simulink model "tqdtqr_rebuild_V3"  (R2021b)
settings: Solver=VariableStepAuto  StartTime=0.0  StopTime=10.0  RelTol=1e-3
undefined symbols (not defined in the file): ATQD_AfterTqMinGain_X_Deg, ATQD_APSCreepBaseTqD_X_kph, ATQD_APSCreepBaseTqD_Y_Deg, ATQD_APSCreepBaseTqR_X_kph, ATQD_APSCreepBaseTqR_Y_Deg, ATQD_APSCreepIterm_X_kph, ATQD_APSCreepIterm_Y_kph, ATQD_APSCreepPterm_X_kph, ATQD_APSCreepPterm_Y_kph, ATQD_APSDecReq_X_kph, ATQD_APSDecReq_Y_mps2, ATQD_APSDecReqCMD_X_kph, ATQD_APSDecReqTs_X_pct, ATQD_APSDecTimeGain_X_Deg, ATQD_APSDecTimeGain_Y_s, ATQD_APSReqLowSpd_X_Deg, ATQD_AutoHoldReleaseBPS_X_Deg, ATQD_AWDLoadTrqnsGain_X_kg, ATQD_AWDLoadTrqnsGain_Y_pct, ATQD_BOSEnBPSPosn_X_kph, ATQD_BOSMap_X_rpm, ATQD_BOSMap_Y_pct, ATQD_CreepBaseTqD_X_kph, ATQD_CreepBaseTqD_Y_Deg, ATQD_CreepBaseTqR_X_kph, ATQD_CreepBaseTqR_Y_Deg, ATQD_CreepBPSDisPosn_X_Deg, ATQD_CreepBPSDisPosnR_X_Deg, ATQD_CreepBPSEnPosn_X_Deg, ATQD_CreepBPSEnPosnR_X_Deg, ATQD_CreepDeltaTq_X_kph, ATQD_CreepIterm_X_kph, ATQD_CreepIterm_Y_kph, ATQD_CreepItermMaxLimit_X_pct, ATQD_CreepPreloadTime_X_kph, ATQD_CreepPreloadTq_X_kph, ATQD_CreepPreloadTq_Y_s, ATQD_CreepProtTq_X_Deg, ATQD_CreepPterm_X_kph, ATQD_CreepPterm_Y_kph, ATQD_CreepRrTqSpRat_X_rpm, ATQD_CreepRrTqSpRat_Y_Nm, ATQD_CreepTargetSpdD_X_pct, ATQD_CreepTargetSpdR_X_pct, ATQD_CreepUpLimitTq_X_rpm, ATQD_DecIneOPDHoldEnDelay_X_Deg, ATQD_DecIneOPDHoldEnDelay_Y_bar, ATQD_ECOTqMapD_X_rpm, ATQD_ECOTqMapD_Y_pct, ATQD_EMTqMapD_X_rpm, ATQD_EMTqMapD_Y_pct, ATQD_EOPDTqMapDCon_X_rpm, ATQD_EOPDTqMapDCon_Y_Deg, ATQD_EstInitVehWeight_X_c, ATQD_FAfterTqCMDGain_X_rpm, ATQD_FAfterTqCMDGain_Y_pct, ATQD_ForceLowSpd_X_Deg, ATQD_ForcePLimitSpd_X_Deg, ATQD_FrLossMAPLowV_X_rpm, ATQD_FrLossMAPLowV_Y_Nm ... (+949)
libraries: simulink x235, hcu_lib x208, tqr x63, tqd x6
(part 28 of 37)

== system tqdtqr_rebuild_V3/Input_Convert/Signal function/SWC1 SWC2 status/SWC2_Subsystem/Road Speed Limit Convert ==
  note: change units and ouput speed
  note: Calculate speed after offset
  note: Calculate road limit speed
  VINP_ADASSLIFSpdLim_enum : Inport
  VINP_IVIISAOffsetSpd_enum : Inport  Port=2
  VTQD_IVIISAOffsetSpdCHOOSE_flg : Inport  Port=3
  VINP_Distanceunit_flg : Inport  Port=4
  VTQD_ShiftGearPosn_enum : Inport  Port=5
  " 20" : Constant  Value=KTQD_ACCActiveMetSpdLoMPH_mph
  " 30kph" : Constant  Value=KTQD_ACCActiveMetSpdLo_kph
  AND{,1..3} (4 alike) : Logic  AllPortsSameDT=off  OutDataTypeStr=boolean
  Add{,1..3} (4 alike) : Sum  Inputs=+-
  Add4 : Sum
  Constant{,17..18,20} (4 alike) : Constant  Value=0x11  OutDataTypeStr=uint8
  Constant1 : Constant  Value=10  OutDataTypeStr=single
  Constant10 : Constant  Value=15  OutDataTypeStr=single
  Constant11 : Constant  Value=ZERO_FLOAT  OutDataTypeStr=single
  Constant12 : Constant  Value=ENUM_GEARPOSNTOCAN_D  OutDataTypeStr=uint8
  Constant13 : Constant  Value=ZERO_FLOAT  OutDataTypeStr=single
  Constant15 : Constant  Value=ZERO_FLOAT  OutDataTypeStr=single
  Constant16 : Constant  Value=KTQD_SpdLimOffsetOn_flg  OutDataTypeStr=single
  Constant19 : Constant  Value=MPH2KPH  OutDataTypeStr=uint8
  Constant2 : Constant  Value=0xF  OutDataTypeStr=uint8
  Constant21 : Constant  Value=KPH2MPH  OutDataTypeStr=uint8
  Constant22 : Constant  Value=0x0  OutDataTypeStr=uint8
  Constant23 : Constant  Value=0x6  OutDataTypeStr=uint8
  Constant24 : Constant  Value=0x7  OutDataTypeStr=uint8
  Constant25 : Constant  Value=0x8  OutDataTypeStr=uint8
  Constant26 : Constant  Value=0xC  OutDataTypeStr=uint8
  Constant{3,7..9} (4 alike) : Constant  Value=5  OutDataTypeStr=single
  Constant4 : Constant  Value=0x0  OutDataTypeStr=uint8
  Constant5 : Constant  Value=0x9  OutDataTypeStr=uint8
  Constant6 : Constant  Value=0x9  OutDataTypeStr=uint8
  Data Type Conversion{,1..3} (4 alike) : DataTypeConversion  OutDataTypeStr=single
  Delay : Delay  DelayLength=1
      settings: AttributesFormatString=%<InitialCondition>
  Divide : Product  Inputs=**
  Divide1 : Product  Inputs=**
  Equal : RelationalOperator  Operator=~=  OutDataTypeStr=boolean  RndMeth=Simplest
  Equal1 : RelationalOperator  Operator===  OutDataTypeStr=boolean  RndMeth=Simplest
  Max : MinMax  Function=max  Inputs=2
  NOT : Logic  Operator=NOT  AllPortsSameDT=off  OutDataTypeStr=boolean
  NOT1 : Logic  Operator=NOT  AllPortsSameDT=off  OutDataTypeStr=boolean
  OR : Logic  Operator=OR  Inputs=5  AllPortsSameDT=off  OutDataTypeStr=boolean
  Product{,1..3} (4 alike) : Product
  Relational Operator{,1,3..5,10} (6 alike) : RelationalOperator  OutDataTypeStr=boolean  RndMeth=Simplest
  Relational Operator{6..9} (4 alike) : RelationalOperator  Operator===  OutDataTypeStr=boolean  RndMeth=Simplest
  Switch{,1..9} (10 alike) : Switch  Criteria=u2 ~= 0
      settings: AttributesFormatString=%<Criteria>
  VTQD_RoadSpdLim_raw32 : Outport
  wires:
  Relational Operator10/1 -> OR/5
  Relational Operator9/1 -> OR/4
  Relational Operator8/1 -> OR/3
  Relational Operator7/1 -> OR/2
  Relational Operator6/1 -> OR/1
  [VINP_IVIISAOffsetSpd_enum] -> Relational Operator10/1
  Constant26/1 -> Relational Operator10/2
  Constant25/1 -> Relational Operator9/2
  [VINP_IVIISAOffsetSpd_enum] -> Relational Operator9/1
  [VINP_IVIISAOffsetSpd_enum] -> Relational Operator8/1
  Constant24/1 -> Relational Operator8/2
  Constant23/1 -> Relational Operator7/2
  [VINP_IVIISAOffsetSpd_enum] -> Relational Operator7/1
  [VINP_IVIISAOffsetSpd_enum] -> Relational Operator6/1
  Constant22/1 -> Relational Operator6/2
  [VTQD_SpdLimAftOffset_raw32] -> Switch9/3
  Divide1/1 -> Switch9/1
  [VTQD_SpdLimAftOffset_raw32] -> Divide1/1
  Constant21/1 -> Divide1/2
  NOT1/1 -> AND3/2
  Switch9/1 -> Switch8/3
  Constant20/1 -> Relational Operator5/2
  [VINP_ADASSLIFSpdLim_enum] -> Relational Operator5/1
  Relational Operator5/1 -> NOT1/1
  [VINP_Distanceunit_flg] -> AND3/1
  AND3/1 -> Switch9/2
  Constant19/1 -> Divide/2
  Divide/1 -> Switch8/1
  [VTQD_SpdLimAftOffset_raw32] -> Divide/1
  NOT/1 -> AND2/1
  Switch8/1 -> Switch7/3
  Constant18/1 -> Relational Operator4/2
  [VINP_ADASSLIFSpdLim_enum] -> Relational Operator4/1
  Relational Operator4/1 -> AND2/2
  [VINP_Distanceunit_flg] -> NOT/1
  AND2/1 -> Switch8/2
  [VTQD_SpdLimAftOffset_raw32] -> Switch7/1
  Switch7/1 -> Max/2
  AND1/1 -> Switch7/2
  [VINP_Distanceunit_flg] -> AND1/1
  Relational Operator3/1 -> AND1/2
  [VINP_ADASSLIFSpdLim_enum] -> Relational Operator3/1
  Constant17/1 -> Relational Operator3/2
  Constant16/1 -> AND/2
  AND/1 -> Switch3/2
  Constant15/1 -> Switch6/1
  OR/1 -> Switch6/2
  [VTQD_CalRoadSpdLimOffSet_c] -> Switch6/3
  [VTQD_ShiftGearPosn_enum] -> Equal1/1
  VTQD_ShiftGearPosn_enum/1 -> [VTQD_ShiftGearPosn_enum]
  Constant13/1 -> Switch5/3
  Switch1/1 -> Switch5/1
  Constant12/1 -> Equal1/2
  Equal1/1 -> Switch5/2
  [VINP_ADASSLIFSpdLim_enum] -> Equal/1
  Add4/1 -> [VTQD_SpdLimAftOffset_raw32]  "VTQD_SpdLimAftOffset_raw32"
  Max/1 -> [VTQD_RoadSpdLim_raw32]  "VTQD_RoadSpdLim_raw32"
  Switch4/1 -> Max/1
  Delay/1 -> Switch1/3
  VINP_Distanceunit_flg/1 -> [VINP_Distanceunit_flg]
  [VINP_Distanceunit_flg] -> Switch4/2
  " 30kph"/1 -> Switch4/3
  " 20"/1 -> Switch4/1
  [VTQD_IVIISAOffsetSpdCHOOSE_flg] -> AND/1
  [VTQD_RoadSpdLim_raw32] -> VTQD_RoadSpdLim_raw32/1
  [VTQD_CalRoadSpdLim_raw32] -> Add4/1
  Switch6/1 -> Add4/2
  Switch3/1 -> [VTQD_CalRoadSpdLimOffSet_c]  "VTQD_CalRoadSpdLimOffSet_c"
  Constant11/1 -> Switch3/3
  Switch2/1 -> Switch3/1
  VTQD_IVIISAOffsetSpdCHOOSE_flg/1 -> [VTQD_IVIISAOffsetSpdCHOOSE_flg]
  Add2/1 -> Switch2/1
  Add3/1 -> Switch2/3
  Product3/1 -> Add3/1
  Constant10/1 -> Add3/2
  Data Type Conversion3/1 -> Product3/1
  Constant9/1 -> Product3/2
  [VINP_IVIISAOffsetSpd_enum] -> Data Type Conversion3/1
  Constant8/1 -> Add2/2
  Product2/1 -> Add2/1
  Constant7/1 -> Product2/2
  Add1/1 -> Data Type Conversion2/1
  Constant6/1 -> Add1/2
  [VINP_IVIISAOffsetSpd_enum] -> Add1/1
  Data Type Conversion2/1 -> Product2/1
  Relational Operator1/1 -> Switch2/2
  Constant5/1 -> Relational Operator1/2
  [VINP_IVIISAOffsetSpd_enum] -> Relational Operator1/1
  Switch5/1 -> Delay/1, [VTQD_CalRoadSpdLim_raw32]  "VTQD_CalRoadSpdLim_raw32"
  Switch/1 -> Switch1/1
  Constant4/1 -> Equal/2
  Equal/1 -> Switch1/2
  Data Type Conversion1/1 -> Product1/1
  Add/1 -> Data Type Conversion1/1
  Constant3/1 -> Product1/2
  Product1/1 -> Switch/1
  Constant2/1 -> Add/2
  [VINP_ADASSLIFSpdLim_enum] -> Add/1
  Product/1 -> Switch/3
  Constant1/1 -> Product/2
  Data Type Conversion/1 -> Product/1
  [VINP_ADASSLIFSpdLim_enum] -> Data Type Conversion/1
  Constant/1 -> Relational Operator/2
  Relational Operator/1 -> Switch/2
  [VINP_ADASSLIFSpdLim_enum] -> Relational Operator/1
  VINP_IVIISAOffsetSpd_enum/1 -> [VINP_IVIISAOffsetSpd_enum]
  VINP_ADASSLIFSpdLim_enum/1 -> [VINP_ADASSLIFSpdLim_enum]

== system tqdtqr_rebuild_V3/Input_Convert/Signal function/SWC1 SWC2 status/SWC2_Subsystem/Speed Setting Mode ==
  note: Ctrl Mode -> speed(ACC/CC/MSA/ISA)
  note: Ctrl Mode -> OUTPUT SET SPEED
  note: Check PWRSTA and DRIVE GEAR GOOD
  note: INPUT Signal
  note: Botton logic
  VPMM_PowerSta_enum : Inport
  VTQD_ShiftGearPosn_enum : Inport  Port=2
  VTQD_SpdCtrlMode_enum : Inport  Port=3
  VINP_ADASACCSta_enum : Inport  Port=4
  VVMC_CCCtrlSta_enum : Inport  Port=5
  VVMC_MSACtrlSta_enum : Inport  Port=6
  VINP_ADASSLIFSpdLim_enum : Inport  Port=7
  VTQD_SWC2ScrollUpSta_flg : Inport  Port=8
  VTQD_SWC2ScrollDownSta_flg : Inport  Port=9
  task_time_s : Inport  Port=10
  VVMC_LVDAACCStatusInformation_flg : Inport  Port=11
  VTQD_SpdLim4SetSpd_raw32 : Inport  Port=12
  VINP_Distanceunit_flg : Inport  Port=13
  VINP_SmartEcoModeSW_flg : Inport  Port=14
  VINP_IVIACCAdaptiveSta_flg : Inport  Port=15
  VTQD_Set2MeterSpd_flg : Inport  Port=16
  VTQD_SetRoadSpdLim_flg : Inport  Port=17
  VTQD_LScrollPressShort_flg : Inport  Port=18
  VVMC_MeterIndSpeed_raw32 : Inport  Port=19
  ACC Speed Setting ON : Subsystem  TreatAsAtomicUnit=on
  AND{1..5} (5 alike) : Logic  AllPortsSameDT=off  OutDataTypeStr=boolean
  CC Speed Setting ON : Subsystem  TreatAsAtomicUnit=on
  Constant : Constant  Value=ZERO_INT
  Constant1 : Constant  Value=ENUM_SPDCTRLMODE_CC
  Constant10 : Constant  Value=ENUM_SPDCTRLMODE_ISA
  Constant11 : Constant  Value=ENUM_SPDCTRLMODE_OFF
  Constant12 : Constant  Value=KTQD_SetSpdDeltaLongFit_kph
  Constant13 : Constant  Value=ZERO_INT
  Constant2 : Constant  Value=ENUM_POWERSTA_READY
  Constant20 : Constant  Value=KTQD_SpdCtrlModeChgHoldTime_s
  Constant21 : Constant  Value=KTQD_SCPMemSpdTest_flg
  Constant3 : Constant  Value=ENUM_SPDCTRLMODE_ACC
  Constant4 : Constant  Value=ENUM_GEARPOSNTOCAN_D
  Constant5 : Constant  Value=ENUM_SPDCTRLMODE_MSA
  Constant6 : Constant  Value=ENUM_SPDCTRLMODE_ISA
  Constant7 : Constant  Value=ENUM_SPDCTRLMODE_ACC
  Constant8 : Constant  Value=ENUM_SPDCTRLMODE_CC
  Constant9 : Constant  Value=ENUM_SPDCTRLMODE_MSA
  Data Type Conversion : DataTypeConversion  OutDataTypeStr=uint8
  Delay : Delay  DelayLength=1
  Delay Enable : hcu_lib/Basic_Blocks/DelayEnable
  Detect Change : simulink/Logic and Bit Operations/Detect Change  vinit=boolean(0)  OutDataTypeStr=boolean
  Detect Change1 : simulink/Logic and Bit Operations/Detect Change  vinit=boolean(0)  OutDataTypeStr=boolean
  Else Speed Setting On : Subsystem  TreatAsAtomicUnit=on
  Equal{1..11} (11 alike) : RelationalOperator  Operator===  OutDataTypeStr=boolean  RndMeth=Simplest
  ISA Speed Setting ON : Subsystem  TreatAsAtomicUnit=on
  If : If  NumInputs=4  IfExpression=u1 ~= 0  ElseIfExpressions=u2 ~= 0, u3~= 0, u4~= 0
  MSA Speed Setting ON : Subsystem  TreatAsAtomicUnit=on
  Rem : Math  Operator=rem  SaturateOnIntegerOverflow=on
  SR_Latch1 : hcu_lib/Basic_Blocks/SR_Latch
  SR_Latch7 : hcu_lib/Basic_Blocks/SR_Latch
  SWC2ScrollDownSta : Subsystem
  SWC2ScrollUpSta : Subsystem
  Switch{,1..4,8} (6 alike) : Switch  Criteria=u2 ~= 0
      settings: AttributesFormatString=%<Criteria>
  Unit Delay : UnitDelay  InitialCondition=single(0)  SampleTime=-1  HasFrameUpgradeWarning=on
      settings: AttributesFormatString=%<InitialCondition>
  Unit Delay1 : UnitDelay  SampleTime=-1  HasFrameUpgradeWarning=on
  Unit Delay2 : UnitDelay  InitialCondition=boolean(0)  SampleTime=-1  HasFrameUpgradeWarning=on
      settings: AttributesFormatString=%<InitialCondition>
  Unit Delay3 : UnitDelay  InitialCondition=single(0.0)  SampleTime=-1  HasFrameUpgradeWarning=on
      settings: AttributesFormatString=%<InitialCondition>
  VTQD_SetSpd_kph : Outport
  VTQD_SWC2ScrollUpSta_enum : Outport  Port=2
  wires:
  AND4/1 -> Switch8/2
  Constant21/1 -> AND4/2
  SR_Latch1/1 -> AND4/1
  Detect Change1/1 -> SR_Latch1/1
  [VTQD_SpdCtrlMode_enum] -> Detect Change1/1
  Unit Delay3/1 -> Switch8/1
  [VTQD_SetSpd_kph] -> Unit Delay3/1
  Switch/1 -> Switch8/3
  Unit Delay2/1 -> SR_Latch7/2
  SR_Latch7/1 -> Delay Enable/1
  Detect Change/1 -> SR_Latch7/1
  Delay Enable/1 -> Unit Delay2/1, SR_Latch1/2
  Constant20/1 -> Delay Enable/2
  [task_time_s] -> Delay Enable/3
  [VTQD_SpdCtrlMode_enum] -> Detect Change/1
  [VTQD_SetSpd_kph] -> Unit Delay1/1
  Unit Delay1/1 -> MSA Speed Setting ON/13(VTQD_LastSetSpd_kph)
  Unit Delay/1 -> ACC Speed Setting ON/16(VTQD_LastSetSpd_kph)
  [VTQD_SetSpd_kph] -> Unit Delay/1
  [VTQD_SWC2ScrollUpSta_flg] -> ACC Speed Setting ON/15(VTQD_SWC2ScrollUpSta_flg)
  [VTQD_SWC2ScrollDownSta_flg] -> ACC Speed Setting ON/14(VTQD_SWC2ScrollDownSta_flg)
  [VVMC_LVDAACCStatusInformation_flg] -> ACC Speed Setting ON/3(VVMC_LVDAACCStatusInformation_flg)
  VVMC_LVDAACCStatusInformation_flg/1 -> [VVMC_LVDAACCStatusInformation_flg]
  [VVMC_MeterIndSpeed_raw32] -> MSA Speed Setting ON/12(VVMC_MeterIndSpeed_raw32)
  [VVMC_MeterIndSpeed_raw32] -> ACC Speed Setting ON/13(VVMC_MeterIndSpeed_raw32)
  VVMC_MeterIndSpeed_raw32/1 -> [VVMC_MeterIndSpeed_raw32]
  [VTQD_LScrollPressShort_flg] -> MSA Speed Setting ON/11(VTQD_LScrollPressShort_flg)
  [VINP_ADASSLIFSpdLim_enum] -> MSA Speed Setting ON/10(VINP_ADASSLIFSpdLim_enum)
  [VTQD_SetRoadSpdLim_flg] -> MSA Speed Setting ON/9(VTQD_SetRoadSpdLim_flg)
  [VTQD_Set2MeterSpd_flg] -> MSA Speed Setting ON/8(VTQD_Set2MeterSpd_flg)
  [VINP_IVIACCAdaptiveSta_flg] -> MSA Speed Setting ON/7(VINP_IVIACCAdaptiveSta_flg)
  VTQD_LScrollPressShort_flg/1 -> [VTQD_LScrollPressShort_flg]
  VTQD_SetRoadSpdLim_flg/1 -> [VTQD_SetRoadSpdLim_flg]
  VTQD_Set2MeterSpd_flg/1 -> [VTQD_Set2MeterSpd_flg]
  [VINP_IVIACCAdaptiveSta_flg] -> ACC Speed Setting ON/8(VINP_IVIACCAdaptiveSta_flg)
  [VTQD_LScrollPressShort_flg] -> ACC Speed Setting ON/12(VTQD_LScrollPressShort_flg)
  [VINP_ADASSLIFSpdLim_enum] -> ACC Speed Setting ON/11(VINP_ADASSLIFSpdLim_enum)
  [VTQD_SetRoadSpdLim_flg] -> ACC Speed Setting ON/10(VTQD_SetRoadSpdLim_flg)
  [VTQD_Set2MeterSpd_flg] -> ACC Speed Setting ON/9(VTQD_Set2MeterSpd_flg)
  VINP_IVIACCAdaptiveSta_flg/1 -> [VINP_IVIACCAdaptiveSta_flg]
  [VINP_SmartEcoModeSW_flg] -> ISA Speed Setting ON/2(VINP_SmartEcoModeSW_flg)
  [VINP_SmartEcoModeSW_flg] -> MSA Speed Setting ON/6(VINP_SmartEcoModeSW_flg)
  [VINP_SmartEcoModeSW_flg] -> CC Speed Setting ON/7(VINP_SmartEcoModeSW_flg)
  [VINP_SmartEcoModeSW_flg] -> ACC Speed Setting ON/7(VINP_SmartEcoModeSW_flg)
  VINP_SmartEcoModeSW_flg/1 -> [VINP_SmartEcoModeSW_flg]
  [VTQD_SWC2ScrollDownSta_enum] -> MSA Speed Setting ON/3("VTQD_SWC2ScrollDownSta_enum  ")
  [VTQD_SWC2ScrollUpSta_enum] -> MSA Speed Setting ON/2("VTQD_SWC2ScrollUpSta_enum  ")
  [VTQD_SWC2ScrollUpSta_enum] -> ACC Speed Setting ON/1(VTQD_SWC2ScrollUpSta_enum)
  [VTQD_SWC2ScrollDownSta_enum] -> ACC Speed Setting ON/2(VTQD_SWC2ScrollDownSta_enum)
  [VINP_Distanceunit_flg] -> MSA Speed Setting ON/5(VINP_Distanceunit_flg)
  [VINP_Distanceunit_flg] -> CC Speed Setting ON/6(VINP_Distanceunit_flg)
  [VINP_Distanceunit_flg] -> ACC Speed Setting ON/6(VINP_Distanceunit_flg)
  VINP_Distanceunit_flg/1 -> [VINP_Distanceunit_flg]
  VTQD_SpdLim4SetSpd_raw32/1 -> [VTQD_SpdLim4SetSpd_raw32]
  ACC Speed Setting ON/1(VTQD_ACCSetSpd_kph) -> [VTQD_ACCSetSpd_kph]  "VTQD_SWC2ACCSetSpd_kph"
  [VTQD_SpdLim4SetSpd_raw32] -> ACC Speed Setting ON/4(VTQD_SpdLim4SetSpd_raw32)
  [VINP_ADASACCSta_enum] -> ACC Speed Setting ON/5(VINP_ADASACCSta_enum)
  [VTQD_ElseSetSpd_kph] -> Switch4/3
  Else Speed Setting On/1(Out) -> [VTQD_ElseSetSpd_kph]
  Constant13/1 -> Else Speed Setting On/1(In)
  [VTQD_SpdLim4SetSpd_raw32] -> MSA Speed Setting ON/4(VTQD_SpdLim4SetSpd_raw32)
  [VTQD_SpdLim4SetSpd_raw32] -> CC Speed Setting ON/4(VTQD_SpdLim4SetSpd_raw32)
  [VTQD_SetSpdDeltaLongFit_kph] -> CC Speed Setting ON/5(VTQD_SetSpdDeltaLongFit_kph)
  Constant12/1 -> Rem/2
  Delay/1 -> Rem/1
  [VTQD_SetSpd_kph] -> Delay/1
  Data Type Conversion/1 -> [VTQD_SetSpdDeltaLongFit_kph]  "VTQD_SetSpdDeltaLongFit_kph"
  Rem/1 -> Data Type Conversion/1
  [task_time_s] -> SWC2ScrollUpSta/2(task_time_s)
  SWC2ScrollDownSta/1(OUTPUT) -> [VTQD_SWC2ScrollDownSta_enum]  "VTQD_SWC2ScrollDownSta_enum"
  [VTQD_SWC2ScrollDownSta_flg] -> SWC2ScrollDownSta/1(INPUT)
  [task_time_s] -> SWC2ScrollDownSta/2(task_time_s)
  SWC2ScrollUpSta/1(OUTPUT) -> [VTQD_SWC2ScrollUpSta_enum]  "VTQD_SWC2ScrollUpSta_enum"
  [VTQD_SWC2ScrollUpSta_flg] -> SWC2ScrollUpSta/1(INPUT)
  [VINP_ADASSLIFSpdLim_enum] -> ISA Speed Setting ON/1(VINP_ADASSLIFSpdLim_enum)
  VPMM_PowerSta_enum/1 -> [VPMM_PowerSta_enum]
  VTQD_ShiftGearPosn_enum/1 -> [VTQD_ShiftGearPosn_enum]
  [VTQD_PwrstaANDGearRdy_flg] -> AND1/1
  VTQD_SpdCtrlMode_enum/1 -> [VTQD_SpdCtrlMode_enum]
  If/1 -> ACC Speed Setting ON/Action
  [VTQD_SpdCtrlMode_enum] -> Equal3/1
  Constant3/1 -> Equal3/2
  Equal3/1 -> AND1/2
  AND1/1 -> If/1
  Equal4/1 -> AND2/2
  Equal2/1 -> AND2/1
  Constant4/1 -> Equal4/2
  [VTQD_ShiftGearPosn_enum] -> Equal4/1
  Constant2/1 -> Equal2/2
  [VPMM_PowerSta_enum] -> Equal2/1
  AND2/1 -> [VTQD_PwrstaANDGearRdy_flg]  "VTQD_PwrstaANDGearRdy_flg"
  Equal1/1 -> AND3/2
  Constant1/1 -> Equal1/2
  [VTQD_SpdCtrlMode_enum] -> Equal1/1
  [VTQD_PwrstaANDGearRdy_flg] -> AND3/1
  AND3/1 -> If/2
  VTQD_SWC2ScrollUpSta_flg/1 -> [VTQD_SWC2ScrollUpSta_flg]
  VTQD_SWC2ScrollDownSta_flg/1 -> [VTQD_SWC2ScrollDownSta_flg]
  VINP_ADASACCSta_enum/1 -> [VINP_ADASACCSta_enum]
  [VVMC_CCCtrlSta_enum] -> CC Speed Setting ON/1(VVMC_CCCtrlSta_enum)
  [VTQD_SWC2ScrollUpSta_enum] -> CC Speed Setting ON/2("VTQD_SWCResUpPress_enum  ")
  [VTQD_SWC2ScrollDownSta_enum] -> CC Speed Setting ON/3("VTQD_SWCSetDownPress_enum  ")
  If/2 -> CC Speed Setting ON/Action
  [VVMC_MSACtrlSta_enum] -> MSA Speed Setting ON/1(VVMC_MSACrlSta_enum)
  If/3 -> MSA Speed Setting ON/Action
  [VTQD_SpdCtrlMode_enum] -> Equal5/1
  Constant5/1 -> Equal5/2
  Equal5/1 -> If/3
  VVMC_MSACtrlSta_enum/1 -> [VVMC_MSACtrlSta_enum]
  Equal6/1 -> AND5/2
  Constant6/1 -> Equal6/2
  [VTQD_SpdCtrlMode_enum] -> Equal6/1
  [VTQD_PwrstaANDGearRdy_flg] -> AND5/1
  AND5/1 -> If/4
  If/4 -> ISA Speed Setting ON/Action
  If/5 -> Else Speed Setting On/Action
  ISA Speed Setting ON/1(VTQD_ISASetSpd_kph) -> [VTQD_ISASetSpd_kph]  "VTQD_SWC2ISASetSpd_kph"
  Constant7/1 -> Equal7/2
  [VTQD_SpdCtrlMode_enum] -> Equal7/1
  Equal7/1 -> Switch/2
  [VTQD_ACCSetSpd_kph] -> Switch/1
  [VTQD_CCSetSpd_kph] -> Switch1/1
  Equal8/1 -> Switch1/2
  [VTQD_SpdCtrlMode_enum] -> Equal8/1
  Constant8/1 -> Equal8/2
  Switch1/1 -> Switch/3
  Constant9/1 -> Equal9/2
  [VTQD_SpdCtrlMode_enum] -> Equal9/1
  Equal9/1 -> Switch2/2
  [VTQD_MSASetSpd_kph] -> Switch2/1
  Switch2/1 -> Switch1/3
  [VTQD_ISASetSpd_kph] -> Switch3/1
  Equal10/1 -> Switch3/2
  [VTQD_SpdCtrlMode_enum] -> Equal10/1
  Constant10/1 -> Equal10/2
  Switch3/1 -> Switch2/3
  Constant11/1 -> Equal11/2
  [VTQD_SpdCtrlMode_enum] -> Equal11/1
  Equal11/1 -> Switch4/2
  Switch4/1 -> Switch3/3
  Constant/1 -> Switch4/1
  Switch8/1 -> [VTQD_SetSpd_kph]  "VTQD_SetSpd_kph"
  task_time_s/1 -> [task_time_s]
  VINP_ADASSLIFSpdLim_enum/1 -> [VINP_ADASSLIFSpdLim_enum]
  VVMC_CCCtrlSta_enum/1 -> [VVMC_CCCtrlSta_enum]
  CC Speed Setting ON/1(VTQD_CCSetSpd_kph) -> [VTQD_CCSetSpd_kph]  "VTQD_SWC2CCSetSpd_kph"
  MSA Speed Setting ON/1(VSCP_MSASetSpd_kph) -> [VTQD_MSASetSpd_kph]  "VTQD_SWC2MSASetSpd_kph"
  [VTQD_SWC2ScrollUpSta_enum] -> VTQD_SWC2ScrollUpSta_enum/1
  [VTQD_SetSpd_kph] -> VTQD_SetSpd_kph/1

== system tqdtqr_rebuild_V3/Input_Convert/Signal function/SWC1 SWC2 status/SWC2_Subsystem/VTQD_IVIISAOffsetSpdCHOOSE_flg ==
  VTQD_IVIISAOffsetSpd_enum : Inport
  Constant : Constant  Value=ENUM_IVIISAOFFSETSPD_MIUNS10KPH
  Constant1 : Constant  Value=ENUM_IVIISAOFFSETSPD_MIUNS5KPH
  Constant2 : Constant  Value=ENUM_IVIISAOFFSETSPD_0KPH
  Constant3 : Constant  Value=ENUM_IVIISAOFFSETSPD_PLUS5KPH
  Constant4 : Constant  Value=ENUM_IVIISAOFFSETSPD_PLUS10KPH
  Constant5 : Constant  Value=ENUM_IVIISAOFFSETSPD_MIUNS5MPH
  Constant6 : Constant  Value=ENUM_IVIISAOFFSETSPD_0MPH
  Constant7 : Constant  Value=ENUM_IVIISAOFFSETSPD_PLUS5MPH
  Constant8 : Constant  Value=TRUE
  Constant9 : Constant  Value=FALSE
  Equal{,1..7} (8 alike) : RelationalOperator  Operator===  OutDataTypeStr=boolean  RndMeth=Simplest
  OR : Logic  Operator=OR  Inputs=8  AllPortsSameDT=off  OutDataTypeStr=boolean
  Switch : Switch  Criteria=u2 ~= 0
      settings: AttributesFormatString=%<Criteria>
  VTQD_IVIISAOffsetSpdCHOOSE_flg : Outport
  wires:
  [VTQD_IVIISAOffsetSpd_enum] -> Equal3/1
  [VTQD_IVIISAOffsetSpd_enum] -> Equal7/1
  [VTQD_IVIISAOffsetSpd_enum] -> Equal5/1
  [VTQD_IVIISAOffsetSpd_enum] -> Equal6/1
  [VTQD_IVIISAOffsetSpd_enum] -> Equal4/1
  [VTQD_IVIISAOffsetSpd_enum] -> Equal2/1
  [VTQD_IVIISAOffsetSpd_enum] -> Equal1/1
  Switch/1 -> VTQD_IVIISAOffsetSpdCHOOSE_flg/1  "VTQD_IVIISAOffsetSpdCHOOSE_flg"
  Constant9/1 -> Switch/3
  Constant8/1 -> Switch/1
  OR/1 -> Switch/2
  Equal7/1 -> OR/8
  Constant7/1 -> Equal7/2
  Constant6/1 -> Equal6/2
  Equal6/1 -> OR/7
  Constant3/1 -> Equal3/2
  Equal3/1 -> OR/4
  Constant4/1 -> Equal4/2
  Equal4/1 -> OR/5
  Equal5/1 -> OR/6
  Constant5/1 -> Equal5/2
  Constant2/1 -> Equal2/2
  Equal2/1 -> OR/3
  Equal1/1 -> OR/2
  Constant1/1 -> Equal1/2
  Equal/1 -> OR/1
  Constant/1 -> Equal/2
  VTQD_IVIISAOffsetSpd_enum/1 -> [VTQD_IVIISAOffsetSpd_enum]
  [VTQD_IVIISAOffsetSpd_enum] -> Equal/1

== system tqdtqr_rebuild_V3/Input_Convert/Signal function/SWC1 SWC2 status/SWC_Subsystem/SpdCtrlBotton Behavior ==
  note: Long press or Short press
  note: If press time more then Long press's limit then go Long press only. Else go short press only. Else if no press.
  SWC_ACC_Sta : Inport
  TASK_TIME : Inport  Port=2
  AND : Logic  AllPortsSameDT=off  OutDataTypeStr=boolean
  Constant10 : Constant  Value=FALSE
  Constant3 : Constant  Value=KTQD_SpdModeShortPLim_s
  Constant7 : Constant  Value=FALSE
  Default 3 sec : Constant  Value=KTQD_SpdModeLongPLim_s
  DelayEnable_LONG_PRESS : hcu_lib/Basic_Blocks/DelayEnable
  DelayEnable_SHORT_PRESS : hcu_lib/Basic_Blocks/DelayEnable
  Detect Decrease1 : simulink/Logic and Bit Operations/Detect Decrease  vinit=boolean(0)  OutDataTypeStr=boolean
  Detect Decrease2 : simulink/Logic and Bit Operations/Detect Decrease  vinit=boolean(0)  OutDataTypeStr=boolean
  Detect Increase : simulink/Logic and Bit Operations/Detect Increase  vinit=boolean(0)  OutDataTypeStr=boolean
  Switch1 : Switch  Criteria=u2 > Threshold
      settings: AttributesFormatString=%<Criteria>
  Switch2 : Switch  Criteria=u2 ~= 0
      settings: AttributesFormatString=%<Criteria>
  VTQD_SpdCtrlShortP_flg : Outport
  "VTQD_SpdCtrlLongP_flg\t" : Outport  Port=2
  wires:
  TASK_TIME/1 -> [TASK_TIME]
  Switch1/1 -> [Long_press]
  Detect Decrease2/1 -> [Short_press_falling_Edge]
  Detect Decrease1/1 -> AND/2
  SWC_ACC_Sta/1 -> [SWC_ACC_Sta]
  Switch2/1 -> VTQD_SpdCtrlShortP_flg/1
  AND/1 -> Switch2/2
  [SWC_ACC_Sta] -> DelayEnable_LONG_PRESS/1, DelayEnable_SHORT_PRESS/1
  [Short_press_falling_Edge] -> Switch2/3
  Constant10/1 -> Switch2/1
  [Long_press] -> Detect Increase/1, Detect Decrease1/1
  [Short_press_falling_Edge] -> AND/1
  DelayEnable_LONG_PRESS/1 -> Switch1/2, Switch1/1
  Constant7/1 -> Switch1/3
  DelayEnable_SHORT_PRESS/1 -> Detect Decrease2/1
  Constant3/1 -> DelayEnable_SHORT_PRESS/2
  [TASK_TIME] -> DelayEnable_SHORT_PRESS/3
  Default 3 sec/1 -> DelayEnable_LONG_PRESS/2
  [TASK_TIME] -> DelayEnable_LONG_PRESS/3
  Detect Increase/1 -> "VTQD_SpdCtrlLongP_flg\t"/1

== system tqdtqr_rebuild_V3/Input_Convert/Signal function/SWC1 SWC2 status/SWC_Subsystem/Speed Setting Mode ==
  note: CtrlMode -> Calculate speed(ACC/CC/MSA/ISA)
  note: CtrlMode -> OUTPUT SET SPEED
  note: Check PWRSTA and DRIVE GEAR GOOD
  note: INPUT Signal
  note: Botton logic(long/short press)
  VPMM_PowerSta_enum : Inport
  VTQD_ShiftGearPosn_enum : Inport  Port=2
  VTQD_SpdCtrlMode_enum : Inport  Port=3
  VINP_ADASACCSta_enum : Inport  Port=4
  VVMC_CCCtrlSta_enum : Inport  Port=5
  VVMC_MSACtrlSta_enum : Inport  Port=6
  VINP_ADASVehSpdLim_kph : Inport  Port=7
  VTQD_SWCResUpSta_flg : Inport  Port=8
  VTQD_SWCSetDownSta_flg : Inport  Port=9
  task_time_s : Inport  Port=10
  VVMC_LVDAACCStatusInformation_flg : Inport  Port=11
  VVMC_ACCObjDist_m : Inport  Port=12
  VVMC_MeterIndSpeed_raw32 : Inport  Port=13
  VINP_Distanceunit_flg : Inport  Port=14
  VINP_SmartEcoModeSW_flg : Inport  Port=15
  VVMC_SetACCDisableAPS_flg : Inport  Port=16
  ACC Speed Setting ON : Subsystem  TreatAsAtomicUnit=on
  AND{1..5} (5 alike) : Logic  AllPortsSameDT=off  OutDataTypeStr=boolean
  CC Speed Setting ON : Subsystem  TreatAsAtomicUnit=on
  Constant : Constant  Value=ZERO_INT
  Constant1 : Constant  Value=ENUM_SPDCTRLMODE_CC
  Constant10 : Constant  Value=ENUM_SPDCTRLMODE_ISA
  Constant11 : Constant  Value=ENUM_SPDCTRLMODE_OFF
  Constant12 : Constant  Value=KTQD_SetSpdDeltaLongFit_kph
  Constant13 : Constant  Value=ZERO_INT
  Constant2 : Constant  Value=ENUM_POWERSTA_READY
  Constant3 : Constant  Value=ENUM_SPDCTRLMODE_ACC
  Constant4 : Constant  Value=ENUM_GEARPOSNTOCAN_D
  Constant5 : Constant  Value=ENUM_SPDCTRLMODE_MSA
  Constant6 : Constant  Value=ENUM_SPDCTRLMODE_ISA
  Constant7 : Constant  Value=ENUM_SPDCTRLMODE_ACC
  Constant8 : Constant  Value=ENUM_SPDCTRLMODE_CC
  Constant9 : Constant  Value=ENUM_SPDCTRLMODE_MSA
  Data Type Conversion : DataTypeConversion  OutDataTypeStr=uint8
  Delay : Delay  DelayLength=1  InitialCondition=single(0.0)
      settings: AttributesFormatString=%<InitialCondition>
  Else Speed Setting On : Subsystem  TreatAsAtomicUnit=on
  Equal{1..11} (11 alike) : RelationalOperator  Operator===  OutDataTypeStr=boolean  RndMeth=Simplest
  ISA Speed Setting ON : Subsystem  TreatAsAtomicUnit=on
  If : If  NumInputs=4  IfExpression=u1 ~= 0  ElseIfExpressions=u2 ~= 0, u3~= 0, u4~= 0
  MSA Speed Setting ON : Subsystem  TreatAsAtomicUnit=on
  Rem : Math  Operator=rem  SaturateOnIntegerOverflow=on
  Switch{,1..4} (5 alike) : Switch  Criteria=u2 ~= 0
      settings: AttributesFormatString=%<Criteria>
  VTQD_SWCResUpPress_enum : Subsystem
  VTQD_SWCSetDownPress_enum : Subsystem
  VTQD_SetSpd_kph : Outport
  wires:
  VVMC_SetACCDisableAPS_flg/1 -> ACC Speed Setting ON/10(VVMC_SetACCDisableAPS_flg)
  [VINP_SmartEcoModeSW_flg] -> ACC Speed Setting ON/9(VINP_SmartEcoModeSW_flg)
  [VINP_SmartEcoModeSW_flg] -> CC Speed Setting ON/7(VINP_SmartEcoModeSW_flg)
  [VINP_SmartEcoModeSW_flg] -> MSA Speed Setting ON/7(VINP_SmartEcoModeSW_flg)
  [VINP_SmartEcoModeSW_flg] -> ISA Speed Setting ON/2(VINP_SmartEcoModeSW_flg)
  VINP_SmartEcoModeSW_flg/1 -> [VINP_SmartEcoModeSW_flg]
  [VINP_Distanceunit_flg] -> MSA Speed Setting ON/6(VINP_Distanceunit_flg)
  [VINP_Distanceunit_flg] -> CC Speed Setting ON/6(VINP_Distanceunit_flg)
  [VINP_Distanceunit_flg] -> ACC Speed Setting ON/8(VINP_Distanceunit_flg)
  VINP_Distanceunit_flg/1 -> [VINP_Distanceunit_flg]
  VVMC_MeterIndSpeed_raw32/1 -> [VVMC_MeterIndSpeed_raw32]
  VVMC_LVDAACCStatusInformation_flg/1 -> ACC Speed Setting ON/4(VVMC_LVDAACCStatusInformation_flg)
  ACC Speed Setting ON/1(VTQD_ACCSetSpd_kph) -> [VTQD_ACCSetSpd_kph]  "VTQD_SWCACCSetSpd_kph"
  [task_time_s] -> ACC Speed Setting ON/3(task_time_s)
  [VVMC_MeterIndSpeed_raw32] -> ACC Speed Setting ON/6(VVMC_MeterIndSpeed_raw32)
  [VTQD_SWCSetDownSta_flg] -> ACC Speed Setting ON/2(VTQD_SWCSetDownSta_flg)
  VVMC_ACCObjDist_m/1 -> ACC Speed Setting ON/5(VVMC_ACCObjDist_m)
  [VTQD_SWCResUpSta_flg] -> ACC Speed Setting ON/1(VTQD_SWCResUpSta_flg)
  [VINP_ADASACCSta_enum] -> ACC Speed Setting ON/7(VINP_ADASACCSta_enum)
  [VTQD_ElseSetSpd_kph] -> Switch4/3
  Else Speed Setting On/1(Out) -> [VTQD_ElseSetSpd_kph]
  Constant13/1 -> Else Speed Setting On/1(In)
  [VTQD_SetSpdDeltaLongFit_kph] -> MSA Speed Setting ON/5(VTQD_SetSpdDeltaLongFit_kph)
  [VVMC_MeterIndSpeed_raw32] -> MSA Speed Setting ON/4(VVMC_MeterIndSpeed_raw32)
  [VVMC_MeterIndSpeed_raw32] -> CC Speed Setting ON/4(VVMC_MeterIndSpeed_raw32)
  [VTQD_SetSpdDeltaLongFit_kph] -> CC Speed Setting ON/5(VTQD_SetSpdDeltaLongFit_kph)
  Constant12/1 -> Rem/2
  Delay/1 -> Rem/1
  [VTQD_SetSpd_kph] -> Delay/1
  Data Type Conversion/1 -> [VTQD_SetSpdDeltaLongFit_kph]  "VTQD_SetSpdDeltaLongFit_kph"
  Rem/1 -> Data Type Conversion/1
  [VTQD_SWCSetDownPress_enum] -> MSA Speed Setting ON/3("VTQD_SWCSetDownPress_enum  ")
  [VTQD_SWCResUpPress_enum] -> MSA Speed Setting ON/2("VTQD_SWCResUpPress_enum  ")
  [task_time_s] -> VTQD_SWCResUpPress_enum/2(task_time_s)
  VTQD_SWCSetDownPress_enum/1(OUTPUT) -> [VTQD_SWCSetDownPress_enum]  "VTQD_SWCSetDownPress_enum"
  [VTQD_SWCSetDownSta_flg] -> VTQD_SWCSetDownPress_enum/1(INPUT)
  [task_time_s] -> VTQD_SWCSetDownPress_enum/2(task_time_s)
  VTQD_SWCResUpPress_enum/1(OUTPUT) -> [VTQD_SWCResUpPress_enum]  "VTQD_SWCResUpPress_enum"
  [VTQD_SWCResUpSta_flg] -> VTQD_SWCResUpPress_enum/1(INPUT)
  [VINP_ADASVehSpdLim_kph] -> ISA Speed Setting ON/1(VINP_ADASVehSpdLim_kph)
  VPMM_PowerSta_enum/1 -> [VPMM_PowerSta_enum]
  VTQD_ShiftGearPosn_enum/1 -> [VTQD_ShiftGearPosn_enum]
  [VTQD_PwrstaANDGearGOOD_flg] -> AND1/1
  VTQD_SpdCtrlMode_enum/1 -> [VTQD_SpdCtrlMode_enum]
  If/1 -> ACC Speed Setting ON/Action
  [VTQD_SpdCtrlMode_enum] -> Equal3/1
  Constant3/1 -> Equal3/2
  Equal3/1 -> AND1/2
  AND1/1 -> If/1
  Equal4/1 -> AND2/2
  Equal2/1 -> AND2/1
  Constant4/1 -> Equal4/2
  [VTQD_ShiftGearPosn_enum] -> Equal4/1
  Constant2/1 -> Equal2/2
  [VPMM_PowerSta_enum] -> Equal2/1
  AND2/1 -> [VTQD_PwrstaANDGearGOOD_flg]
  Equal1/1 -> AND3/2
  Constant1/1 -> Equal1/2
  [VTQD_SpdCtrlMode_enum] -> Equal1/1
  [VTQD_PwrstaANDGearGOOD_flg] -> AND3/1
  AND3/1 -> If/2
  VTQD_SWCResUpSta_flg/1 -> [VTQD_SWCResUpSta_flg]
  VTQD_SWCSetDownSta_flg/1 -> [VTQD_SWCSetDownSta_flg]
  VINP_ADASACCSta_enum/1 -> [VINP_ADASACCSta_enum]
  [VVMC_CCCtrlSta_enum] -> CC Speed Setting ON/1(VVMC_CCCtrlSta_enum)
  [VTQD_SWCResUpPress_enum] -> CC Speed Setting ON/2("VTQD_SWCResUpPress_enum  ")
  [VTQD_SWCSetDownPress_enum] -> CC Speed Setting ON/3("VTQD_SWCSetDownPress_enum  ")
  If/2 -> CC Speed Setting ON/Action
  [VVMC_MSACtrlSta_enum] -> MSA Speed Setting ON/1(VVMC_MSACrlSta_enum)
  If/3 -> MSA Speed Setting ON/Action
  [VTQD_PwrstaANDGearGOOD_flg] -> AND4/1
  [VTQD_SpdCtrlMode_enum] -> Equal5/1
  Constant5/1 -> Equal5/2
  Equal5/1 -> AND4/2
  AND4/1 -> If/3
  VVMC_MSACtrlSta_enum/1 -> [VVMC_MSACtrlSta_enum]
  Equal6/1 -> AND5/2
  Constant6/1 -> Equal6/2
  [VTQD_SpdCtrlMode_enum] -> Equal6/1
  [VTQD_PwrstaANDGearGOOD_flg] -> AND5/1
  AND5/1 -> If/4
  If/4 -> ISA Speed Setting ON/Action
  If/5 -> Else Speed Setting On/Action
  ISA Speed Setting ON/1(VTQD_ISASetSpd_kph) -> [VTQD_ISASetSpd_kph]  "VTQD_SWCISASetSpd_kph"
  Constant7/1 -> Equal7/2
  [VTQD_SpdCtrlMode_enum] -> Equal7/1
  Equal7/1 -> Switch/2
  [VTQD_ACCSetSpd_kph] -> Switch/1
  [VTQD_CCSetSpd_kph] -> Switch1/1
  Equal8/1 -> Switch1/2
  [VTQD_SpdCtrlMode_enum] -> Equal8/1
  Constant8/1 -> Equal8/2
  Switch1/1 -> Switch/3
  Constant9/1 -> Equal9/2
  [VTQD_SpdCtrlMode_enum] -> Equal9/1
  Equal9/1 -> Switch2/2
  [VTQD_MSASetSpd_kph] -> Switch2/1
  Switch2/1 -> Switch1/3
  [VTQD_ISASetSpd_kph] -> Switch3/1
  Equal10/1 -> Switch3/2
  [VTQD_SpdCtrlMode_enum] -> Equal10/1
  Constant10/1 -> Equal10/2
  Switch3/1 -> Switch2/3
  Constant11/1 -> Equal11/2
  [VTQD_SpdCtrlMode_enum] -> Equal11/1
  Equal11/1 -> Switch4/2
  Switch4/1 -> Switch3/3
  Constant/1 -> Switch4/1
  Switch/1 -> [VTQD_SetSpd_kph]
  task_time_s/1 -> [task_time_s]
  VINP_ADASVehSpdLim_kph/1 -> [VINP_ADASVehSpdLim_kph]
  VVMC_CCCtrlSta_enum/1 -> [VVMC_CCCtrlSta_enum]
  CC Speed Setting ON/1(VTQD_CCSetSpd_kph) -> [VTQD_CCSetSpd_kph]  "VTQD_SWCCCSetSpd_kph"
  MSA Speed Setting ON/1(VSCP_MSASetSpd_kph) -> [VTQD_MSASetSpd_kph]  "VTQD_SWCMSASetSpd_kph"
  [VTQD_SetSpd_kph] -> VTQD_SetSpd_kph/1

== system tqdtqr_rebuild_V3/Input_Convert/Signal function/SWC1 SWC2 status/SWC_Subsystem/VTQD_IVIISAOffsetSpdCHOOSE_flg ==
  VTQD_IVIISAOffsetSpd_enum : Inport
  Constant : Constant  Value=ENUM_IVIISAOFFSETSPD_MIUNS10KPH
  Constant1 : Constant  Value=ENUM_IVIISAOFFSETSPD_MIUNS5KPH
  Constant2 : Constant  Value=ENUM_IVIISAOFFSETSPD_0KPH
  Constant3 : Constant  Value=ENUM_IVIISAOFFSETSPD_PLUS5KPH
  Constant4 : Constant  Value=ENUM_IVIISAOFFSETSPD_PLUS10KPH
  Constant5 : Constant  Value=ENUM_IVIISAOFFSETSPD_MIUNS5MPH
  Constant6 : Constant  Value=ENUM_IVIISAOFFSETSPD_0MPH
  Constant7 : Constant  Value=ENUM_IVIISAOFFSETSPD_PLUS5MPH
  Constant8 : Constant  Value=TRUE
  Constant9 : Constant  Value=FALSE
  Equal{,1..7} (8 alike) : RelationalOperator  Operator===  OutDataTypeStr=boolean  RndMeth=Simplest
  OR : Logic  Operator=OR  Inputs=8  AllPortsSameDT=off  OutDataTypeStr=boolean
  Switch : Switch  Criteria=u2 ~= 0
      settings: AttributesFormatString=%<Criteria>
  VTQD_IVIISAOffsetSpdCHOOSE_flg : Outport
  wires:
  [VTQD_IVIISAOffsetSpd_enum] -> Equal3/1
  [VTQD_IVIISAOffsetSpd_enum] -> Equal7/1
  [VTQD_IVIISAOffsetSpd_enum] -> Equal5/1
  [VTQD_IVIISAOffsetSpd_enum] -> Equal6/1
  [VTQD_IVIISAOffsetSpd_enum] -> Equal4/1
  [VTQD_IVIISAOffsetSpd_enum] -> Equal2/1
  [VTQD_IVIISAOffsetSpd_enum] -> Equal1/1
  Switch/1 -> VTQD_IVIISAOffsetSpdCHOOSE_flg/1  "VTQD_IVIISAOffsetSpdCHOOSE_flg"
  Constant9/1 -> Switch/3
  Constant8/1 -> Switch/1
  OR/1 -> Switch/2
  Equal7/1 -> OR/8
  Constant7/1 -> Equal7/2
  Constant6/1 -> Equal6/2
  Equal6/1 -> OR/7
  Constant3/1 -> Equal3/2
  Equal3/1 -> OR/4
  Constant4/1 -> Equal4/2
  Equal4/1 -> OR/5
  Equal5/1 -> OR/6
  Constant5/1 -> Equal5/2
  Constant2/1 -> Equal2/2
  Equal2/1 -> OR/3
  Equal1/1 -> OR/2
  Constant1/1 -> Equal1/2
  Equal/1 -> OR/1
  Constant/1 -> Equal/2
  VTQD_IVIISAOffsetSpd_enum/1 -> [VTQD_IVIISAOffsetSpd_enum]
  [VTQD_IVIISAOffsetSpd_enum] -> Equal/1

== system tqdtqr_rebuild_V3/Input_Convert/Signal function/ShiftModule/Gear Shift Posn Cmd/Drive Protection ==
  VTQD_ShifterHandleCmd_enum : Inport
  VTQD_GearActualPosn_enum : Inport  Port=2
  VTQD_VehActSpd_kph : Inport  Port=3
  VTQD_AfterAvailableTqDemFr_Nm : Inport  Port=4
  VTQR_NoABSREDUWhlTqReq_Nm : Inport  Port=5
  VTQR_NoABSFEDUWhlTqReq_Nm : Inport  Port=6
  VTQD_AfterAvailableTqDemRr_Nm : Inport  Port=7
  task_time_s : Inport  Port=8
  VTQD_BrkSwSta_flg : Inport  Port=9
  AND : Logic  Inputs=6  AllPortsSameDT=off  OutDataTypeStr=boolean
  AND2 : Logic  Inputs=3  AllPortsSameDT=off  OutDataTypeStr=boolean
  AND4 : Logic  AllPortsSameDT=off  OutDataTypeStr=boolean
  Abs{,1,3..4} (4 alike) : Abs
  Constant{3,6..7,10} (4 alike) : Constant  Value=KTQD_DrivProtEnToNTq_Nm
  Constant12 : Constant  Value=ENUM_SHIFTCOMMAND_N
  Constant13 : Constant  Value=KTQD_DriveProtVehSpdGain_kph
  Constant14 : Constant  Value=KTQD_DriveProtVehSpdGain_kph
  Constant16 : Constant  Value=KTQD_DrivProtEnSW_flg
  Constant17 : Constant  Value=KTQD_DriveProtDetTime_s
  Constant4 : Constant  Value=ENUM_GEARACTUALPOSN_D
  Delay{4..8} (5 alike) : Delay  DelayLength=1
  DelayEnable : hcu_lib/Basic_Blocks/DelayEnable
  Equal{,2,6..7} (4 alike) : RelationalOperator  Operator=<=  OutDataTypeStr=boolean  RndMeth=Simplest
  Equal3 : RelationalOperator  Operator===  OutDataTypeStr=boolean  RndMeth=Simplest
  Equal8 : RelationalOperator  Operator===  OutDataTypeStr=boolean  RndMeth=Simplest
  NOT1 : Logic  Operator=NOT  AllPortsSameDT=off  OutDataTypeStr=boolean
  OR1 : Logic  Operator=OR  AllPortsSameDT=off  OutDataTypeStr=boolean
  Relational Operator3 : RelationalOperator  Operator=>  OutDataTypeStr=boolean  RndMeth=Simplest
  Relational Operator4 : RelationalOperator  Operator=<=  OutDataTypeStr=boolean  RndMeth=Simplest
  VTQD_DriveProtRemove_flg : Outport
  VTQD_DriveProtToPsnN_flg : Outport  Port=2
  VTQD_DriveProtEn_flg : Outport  Port=3
  wires:
  [VTQD_DriveProtRemove_flg] -> AND/1
  Delay8/1 -> Equal3/1
  Abs4/1 -> Equal7/1
  Abs3/1 -> Equal6/1
  [VTQD_GearActualPosn_enum] -> Delay8/1
  Abs1/1 -> Equal2/1
  Abs/1 -> Equal/1
  AND2/1 -> [VTQD_DriveProtEn_flg], DelayEnable/1  "VTQD_DriveProtEn_flg"
  Constant3/1 -> Equal/2
  Constant10/1 -> Equal2/2
  Constant6/1 -> Equal6/2
  Constant7/1 -> Equal7/2
  DelayEnable/1 -> [VTQD_DriveProtRemove_flg]  "VTQD_DriveProtRemove_flg"
  [task_time_s] -> DelayEnable/3
  Constant17/1 -> DelayEnable/2
  Constant16/1 -> AND2/2
  Equal8/1 -> AND2/1
  [VTQD_VehActSpd_kph] -> Relational Operator3/1
  Constant14/1 -> Relational Operator3/2
  Constant12/1 -> Equal8/2
  [VTQD_ShifterHandleCmd_enum] -> Equal8/1
  AND/1 -> [VTQD_DriveProtToPsnN_flg]  "VTQD_DriveProtToPsnN_flg"
  Delay7/1 -> [VTQD_AfterAvailableTqDemFr_Nm]
  Delay6/1 -> [VTQR_NoABSREDUWhlTqReq_Nm]
  Delay5/1 -> [VTQR_NoABSFEDUWhlTqReq_Nm]
  VTQR_NoABSFEDUWhlTqReq_Nm/1 -> Delay5/1
  Delay4/1 -> [VTQD_AfterAvailableTqDemRr_Nm]
  task_time_s/1 -> [task_time_s]
  VTQD_AfterAvailableTqDemRr_Nm/1 -> Delay4/1
  Equal7/1 -> AND/6
  [VTQD_AfterAvailableTqDemFr_Nm] -> Abs4/1
  Equal6/1 -> AND/5
  [VTQR_NoABSFEDUWhlTqReq_Nm] -> Abs3/1
  [VTQD_DriveProtToPsnN_flg] -> VTQD_DriveProtToPsnN_flg/1
  VTQR_NoABSREDUWhlTqReq_Nm/1 -> Delay6/1
  VTQD_AfterAvailableTqDemFr_Nm/1 -> Delay7/1
  VTQD_VehActSpd_kph/1 -> [VTQD_VehActSpd_kph]
  VTQD_GearActualPosn_enum/1 -> [VTQD_GearActualPosn_enum]
  VTQD_ShifterHandleCmd_enum/1 -> [VTQD_ShifterHandleCmd_enum]
  Constant4/1 -> Equal3/2
  Equal3/1 -> AND/4
  [VTQR_NoABSREDUWhlTqReq_Nm] -> Abs1/1
  Equal2/1 -> AND/3
  Equal/1 -> AND/2
  [VTQD_AfterAvailableTqDemRr_Nm] -> Abs/1
  [VTQD_DriveProtRemove_flg] -> VTQD_DriveProtRemove_flg/1
  OR1/1 -> AND2/3
  Relational Operator3/1 -> OR1/1
  Constant13/1 -> Relational Operator4/2
  [VTQD_VehActSpd_kph] -> Relational Operator4/1
  Relational Operator4/1 -> AND4/1
  AND4/1 -> OR1/2
  [VTQD_BrkSwSta_flg] -> NOT1/1
  NOT1/1 -> AND4/2
  VTQD_BrkSwSta_flg/1 -> [VTQD_BrkSwSta_flg]
  [VTQD_DriveProtEn_flg] -> VTQD_DriveProtEn_flg/1

== system tqdtqr_rebuild_V3/Input_Convert/Signal function/VehWeightEst/Calaulation/Front Wheel Torque ==
  VINP_FrEDURealTMTq_Nm : Inport
  VTQD_VehWeightEstEn_flg : Inport  Port=2
  VTQD_VehWeightEstDis_flg : Inport  Port=3
  VTQD_VehWeightEstEnd_flg : Inport  Port=4
  task_time_s : Inport  Port=5
  AND : Logic  AllPortsSameDT=off  OutDataTypeStr=boolean
  AND1 : Logic  AllPortsSameDT=off  OutDataTypeStr=boolean
  AND2 : Logic  AllPortsSameDT=off  OutDataTypeStr=boolean
  Abs : Abs
  Add : Sum
  Add1 : Sum
  Add2 : Sum  Inputs=+-
  Constant1 : Constant  Value=ZERO_FLOAT
  Constant2 : Constant  Value=KTQD_VehWeighEstTime_s
  Constant3 : Constant  Value=ZERO_FLOAT
  Constant4 : Constant  Value=KTQD_VehWeighEstTimeTune_cnt
  Constant5 : Constant  Value=ZERO_FLOAT
  Constant6 : Constant  Value=KTQD_EstFrWhlTqDev_Nm
  Data Type Conversion : DataTypeConversion  OutDataTypeStr=uint8
  Delay : Delay  DelayLength=1  InitialCondition=boolean(0)
      settings: AttributesFormatString=%<InitialCondition>
  Delay1 : Delay  DelayLength=1
  Delay2 : Delay  DelayLength=1  InitialCondition=single(0.0)
      settings: AttributesFormatString=%<InitialCondition>
  Delay3 : Delay  DelayLength=1  InitialCondition=boolean(0)
      settings: AttributesFormatString=%<InitialCondition>
  Delay4 : Delay  DelayLength=1  InitialCondition=single(0.0)
      settings: AttributesFormatString=%<InitialCondition>
  Detect Decrease : simulink/Logic and Bit Operations/Detect Decrease  vinit=0.0  OutDataTypeStr=boolean
  Detect Increase : simulink/Logic and Bit Operations/Detect Increase  vinit=0.0  OutDataTypeStr=boolean
  Divide : Product  Inputs=*/
  Divide1 : Product  Inputs=*/
  Min : MinMax  Inputs=2
  NOT : Logic  Operator=NOT  AllPortsSameDT=off  OutDataTypeStr=boolean
  NOT1 : Logic  Operator=NOT  AllPortsSameDT=off  OutDataTypeStr=boolean
  Relational Operator : RelationalOperator  Operator=<=  OutDataTypeStr=boolean  RndMeth=Simplest
  Switch{,1..3} (4 alike) : Switch  Criteria=u2 ~= 0
      settings: AttributesFormatString=%<Criteria>
  Terminator : Terminator
  VTQD_EstFrRealTqAvg_Nm : Outport
  VTQD_EstFrRealTqCheckPass_flg : Outport  Port=2
  wires:
  task_time_s/1 -> [task_time_s]
  VTQD_VehWeightEstEnd_flg/1 -> Terminator/1
  VTQD_VehWeightEstDis_flg/1 -> [VTQD_VehWeightEstDis_flg]
  VTQD_VehWeightEstEn_flg/1 -> [VTQD_VehWeightEstEn_flg]
  VINP_FrEDURealTMTq_Nm/1 -> [VINP_FrEDURealTMTq_Nm]
  AND1/1 -> [VTQD_EstFrRealTqCheckPass_flg]  "VTQD_EstFrRealTqCheckPass_flg"
  [VTQD_VehWeightEstDis_flg] -> AND1/1
  Add2/1 -> Abs/1
  Abs/1 -> Relational Operator/1
  Delay/1 -> NOT/1
  Detect Increase/1 -> Switch2/2
  [task_time_s] -> Divide/2
  [VTQD_EstFrRealTqMin_Nm] -> Delay2/1
  Delay2/1 -> Min/2
  [VTQD_VehWeightEstDis_flg] -> Delay/1
  [VTQD_EstFrRealTqMin_Nm] -> Add2/2
  Constant2/1 -> Divide/1
  Switch2/1 -> Delay4/1, [VTQD_EstFrRealTqMin_Nm]  "VTQD_EstFrRealTqMin_Nm"
  Add1/1 -> Divide1/2  "VTQD_EstCycleCount_cnt"
  Switch1/1 -> Delay1/1, [VTQD_EstFrRealTqSum_Nm]  "VTQD_EstFrRealTqSum_Nm"
  Constant5/1 -> Switch1/1
  NOT/1 -> AND/2
  [VINP_FrEDURealTMTq_Nm] -> Switch/1
  [VTQD_EstFrRealTqAvg_Nm] -> Add2/1
  Constant6/1 -> Relational Operator/2
  Add/1 -> Switch1/3
  Relational Operator/1 -> AND1/2
  [VTQD_VehWeightEstEn_flg] -> Detect Increase/1
  Constant1/1 -> Switch/3
  AND/1 -> Switch/2
  [VTQD_VehWeightEstEn_flg] -> Detect Decrease/1
  [VTQD_EstFrRealTqSum_Nm] -> Divide1/1
  Divide/1 -> Data Type Conversion/1
  Switch/1 -> Add/1
  Divide1/1 -> [VTQD_EstFrRealTqAvg_Nm]  "VTQD_EstFrRealTqAvg_Nm"
  [VTQD_VehWeightEstEn_flg] -> AND/1
  Constant3/1 -> Switch2/1
  Delay1/1 -> Add/2
  [VINP_FrEDURealTMTq_Nm] -> Min/1
  Constant4/1 -> Add1/2
  [VTQD_EstFrRealTqCheckPass_flg] -> VTQD_EstFrRealTqCheckPass_flg/1
  [VTQD_EstFrRealTqAvg_Nm] -> VTQD_EstFrRealTqAvg_Nm/1
  Data Type Conversion/1 -> Add1/1
  Delay3/1 -> NOT1/1
  [VTQD_VehWeightEstEn_flg] -> AND2/1
  AND2/1 -> Switch3/2
  NOT1/1 -> AND2/2
  [VTQD_VehWeightEstDis_flg] -> Delay3/1
  Delay4/1 -> Switch3/3
  Min/1 -> Switch3/1
  Switch3/1 -> Switch2/3
  Detect Decrease/1 -> Switch1/2

== system tqdtqr_rebuild_V3/Input_Convert/Signal function/VehWeightEst/Calaulation/Long Acc ==
  VVMC_LongAcc_Gps : Inport
  VTQD_VehWeightEstEn_flg : Inport  Port=2
  VTQD_VehWeightEstDis_flg : Inport  Port=3
  VTQD_VehWeightEstEnd_flg : Inport  Port=4
  task_time_s : Inport  Port=5
  AND : Logic  AllPortsSameDT=off  OutDataTypeStr=boolean
  AND1 : Logic  AllPortsSameDT=off  OutDataTypeStr=boolean
  AND2 : Logic  AllPortsSameDT=off  OutDataTypeStr=boolean
  Abs : Abs
  Abs1 : Abs
  Add : Sum
  Add1 : Sum
  Add2 : Sum  Inputs=+-
  Constant1 : Constant  Value=ZERO_FLOAT
  Constant2 : Constant  Value=KTQD_VehWeighEstTime_s
  Constant3 : Constant  Value=ZERO_FLOAT
  Constant4 : Constant  Value=KTQD_VehWeighEstTimeTune_cnt
  Constant5 : Constant  Value=ZERO_FLOAT
  Constant6 : Constant  Value=KTQD_EstLongAccDev_Gps
  Constant7 : Constant  Value=KTQD_VehWeighEstIntAcc_Gps
  Constant8 : Constant  Value=KTQD_VehWeighEstIntAcc_Gps
  Data Type Conversion : DataTypeConversion  OutDataTypeStr=uint8
  Delay : Delay  DelayLength=1  InitialCondition=boolean(0)
      settings: AttributesFormatString=%<InitialCondition>
  Delay1 : Delay  DelayLength=1  InitialCondition=single(0.0)
      settings: AttributesFormatString=%<InitialCondition>
  Delay2 : Delay  DelayLength=1  InitialCondition=single(0.0)
      settings: AttributesFormatString=%<InitialCondition>
  Delay3 : Delay  DelayLength=1  InitialCondition=boolean(0)
      settings: AttributesFormatString=%<InitialCondition>
  Delay4 : Delay  DelayLength=1  InitialCondition=single(0.0)
      settings: AttributesFormatString=%<InitialCondition>
  Detect Decrease : simulink/Logic and Bit Operations/Detect Decrease  vinit=boolean(0)  OutDataTypeStr=boolean
  Detect Increase : simulink/Logic and Bit Operations/Detect Increase  vinit=boolean(0)  OutDataTypeStr=boolean
  Divide : Product  Inputs=*/
  Divide1 : Product  Inputs=*/
  Min : MinMax  Inputs=2
  NOT : Logic  Operator=NOT  AllPortsSameDT=off  OutDataTypeStr=boolean
  NOT1 : Logic  Operator=NOT  AllPortsSameDT=off  OutDataTypeStr=boolean
  Relational Operator : RelationalOperator  Operator=<=  OutDataTypeStr=boolean  RndMeth=Simplest
  Relational Operator1 : RelationalOperator  Operator=<=  OutDataTypeStr=boolean  RndMeth=Simplest
  Switch : Switch  Criteria=u2 > Threshold
  Switch1 : Switch  Criteria=u2 > Threshold
  Switch2 : Switch  Criteria=u2 ~= 0
      settings: AttributesFormatString=%<Criteria>
  Switch3 : Switch  Criteria=u2 ~= 0
      settings: AttributesFormatString=%<Criteria>
  Switch4 : Switch  Criteria=u2 ~= 0
      settings: AttributesFormatString=%<Criteria>
  Terminator : Terminator
  VTQD_EstLongAccAvg_Gps : Outport
  VTQD_EstLongAccCheckPass_flg : Outport  Port=2
  wires:
  Constant4/1 -> Add1/2
  [VVMC_LongAcc_Gps] -> Min/1
  Delay1/1 -> Add/2
  Constant3/1 -> Switch2/1
  [VTQD_VehWeightEstEn_flg] -> AND/1
  Divide1/1 -> [VTQD_EstLongAccAvg_Gps]  "VTQD_EstLongAccAvg_Gps"
  Switch/1 -> Add/1
  Data Type Conversion/1 -> Add1/1
  AND/1 -> Switch/2
  Constant1/1 -> Switch/3
  [VTQD_VehWeightEstEn_flg] -> Detect Increase/1
  Relational Operator/1 -> AND1/2
  Divide/1 -> Data Type Conversion/1
  Add/1 -> Switch1/3
  Constant6/1 -> Relational Operator/2
  [VTQD_EstLongAccAvg_Gps] -> Add2/1
  [VVMC_LongAcc_Gps] -> Switch/1
  NOT/1 -> AND/2
  Constant5/1 -> Switch1/1
  Switch1/1 -> [VTQD_EstLongAccSum_Gps], Delay1/1  "VTQD_EstLongAccSum_Gps"
  Add1/1 -> Divide1/2  "VTQD_EstCycleCount_cnt"
  Switch2/1 -> Delay4/1, [VTQD_EstLongAccMin_Gps]  "VTQD_EstLongAccMin_Gps"
  Constant2/1 -> Divide/1
  [VTQD_EstLongAccMin_Gps] -> Add2/2
  [VTQD_VehWeightEstDis_flg] -> Delay/1
  Delay2/1 -> Min/2
  [VTQD_EstLongAccMin_Gps] -> Delay2/1
  [task_time_s] -> Divide/2
  Detect Increase/1 -> Switch2/2
  Delay/1 -> NOT/1
  Abs/1 -> Relational Operator/1
  Add2/1 -> Abs/1
  [VTQD_VehWeightEstDis_flg] -> AND1/1
  AND1/1 -> [VTQD_EstLongAccCheckPass_flg]  "VTQD_EstLongAccCheckPass_flg"
  VVMC_LongAcc_Gps/1 -> [VVMC_LongAcc_Gps]
  VTQD_VehWeightEstEn_flg/1 -> [VTQD_VehWeightEstEn_flg]
  VTQD_VehWeightEstDis_flg/1 -> [VTQD_VehWeightEstDis_flg]
  VTQD_VehWeightEstEnd_flg/1 -> Terminator/1
  task_time_s/1 -> [task_time_s]
  [VTQD_EstLongAccAvg_Gps] -> VTQD_EstLongAccAvg_Gps/1
  [VTQD_EstLongAccCheckPass_flg] -> VTQD_EstLongAccCheckPass_flg/1
  AND2/1 -> Switch3/2
  [VTQD_VehWeightEstDis_flg] -> Delay3/1
  NOT1/1 -> AND2/2
  [VTQD_VehWeightEstEn_flg] -> AND2/1
  Delay3/1 -> NOT1/1
  Min/1 -> Switch3/1
  Delay4/1 -> Switch3/3
  Switch3/1 -> Switch2/3
  Detect Decrease/1 -> Switch1/2
  [VTQD_VehWeightEstEn_flg] -> Detect Decrease/1
  [VTQD_EstLongAccSum_Gps] -> Switch4/3
  Switch4/1 -> Divide1/1
  [VTQD_EstLongAccSum_Gps] -> Abs1/1
  Abs1/1 -> Relational Operator1/1
  Relational Operator1/1 -> Switch4/2
  Constant7/1 -> Relational Operator1/2
  Constant8/1 -> Switch4/1
